simulink model "AEBsystem"  (R2024a)
settings: Solver=VariableStepAuto  StartTime=0.0  StopTime=15  RelTol=1e-3
InitFcn:
  | INITAEB
values from neighbouring files (symbols this model uses):
  conducteurActive_var = Simulink.Parameter    [INITAEB.m]
  decelConducteur = 1.5    [INITAEB.m]
  FFORT_decel = 5.0    (= 5)    [INITAEB.m]
  headwayOffset = 1.0    (= 1)    [INITAEB.m]
  PB1_decel = 1.8    [INITAEB.m]
  PB2_decel = 3.2    [INITAEB.m]
  timeMargin = 0.3    [INITAEB.m]
libraries: simulink x4, sim3dautolib x2, sim3dlib x1
(part 2 of 2)

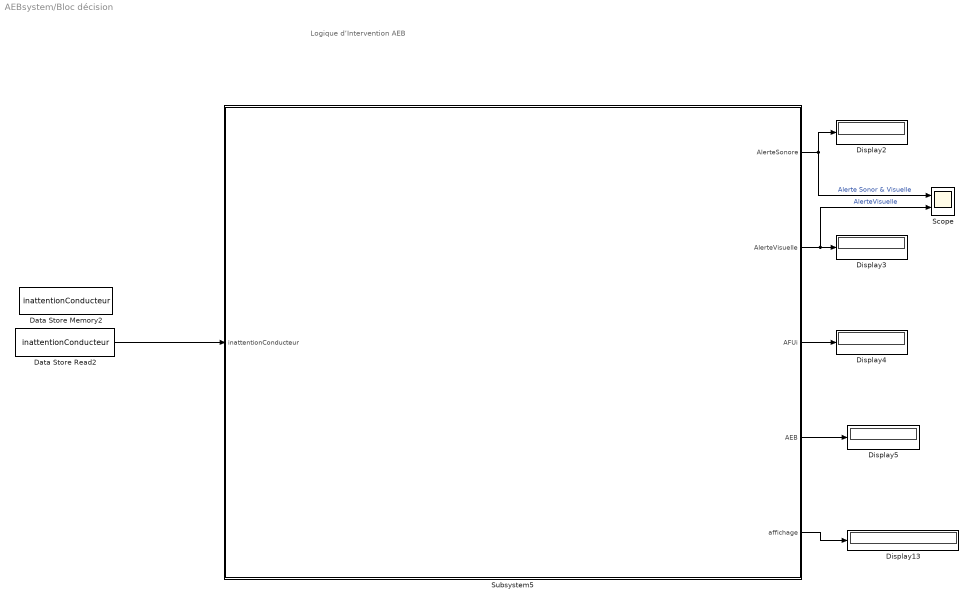
== system AEBsystem/Bloc décision  ==
  note: Logique d’Intervention AEB
  Data Store Memory2 : DataStoreMemory  DataStoreName=inattentionConducteur  WriteAfterWriteMsg=warning  ShowAdditionalParam=off
  Data Store Read2 : DataStoreRead  DataStoreName=inattentionConducteur  IndexOptions=Index vector (dialog)  Indices=1  OutputSizes=1
  Display{2..5,13} (5 alike) : Display
  Scope : Scope  NumInputPorts=2
  Subsystem5 : Subsystem
  wires:
  Subsystem5/1(AlerteSonore) -> Display2/1, Scope/1  "Alerte Sonor & Visuelle"
  Subsystem5/3(AFUi) -> Display4/1
  Subsystem5/2(AlerteVisuelle) -> Scope/2, Display3/1  "AlerteVisuelle"
  Data Store Read2/1 -> Subsystem5/1(inattentionConducteur)
  Subsystem5/4(AEB) -> Display5/1
  Subsystem5/5(affichage) -> Display13/1

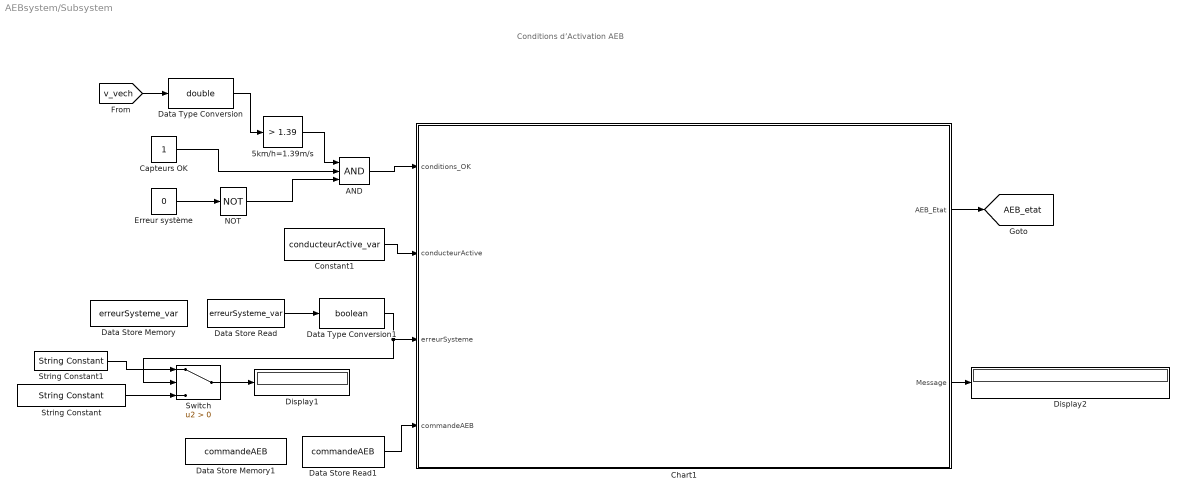
== system AEBsystem/Subsystem ==
  note: Conditions d’Activation AEB
  5km/h=1.39m/s : simulink/Logic and Bit Operations/Compare To Constant  relop=>  const=1.39  OutDataTypeStr=uint8
  AND : Logic  Inputs=3  IconShape=distinctive  AllPortsSameDT=off  OutDataTypeStr=boolean
  Capteurs OK : Constant
  Chart1 : Stateflow chart  TreatAsAtomicUnit=on
  Constant1 : Constant  Value=conducteurActive_var
  Data Store Memory : DataStoreMemory  DataStoreName=erreurSysteme_var  WriteAfterWriteMsg=warning  ShowAdditionalParam=off
  Data Store Memory1 : DataStoreMemory  DataStoreName=commandeAEB  WriteAfterWriteMsg=warning  InitialValue=1  ShowAdditionalParam=off
  Data Store Read : DataStoreRead  DataStoreName=erreurSysteme_var  IndexOptions=Index vector (dialog)  Indices=1  OutputSizes=1
  Data Store Read1 : DataStoreRead  DataStoreName=commandeAEB  IndexOptions=Index vector (dialog)  Indices=1  OutputSizes=1
  Data Type Conversion : DataTypeConversion  OutDataTypeStr=double  SaturateOnIntegerOverflow=off  RndMeth=Floor
  Data Type Conversion1 : DataTypeConversion  OutDataTypeStr=boolean  SaturateOnIntegerOverflow=off  RndMeth=Floor
  Display1 : Display
  Display2 : Display
  Erreur système : Constant  Value=0
  NOT : Logic  Operator=NOT  IconShape=distinctive  AllPortsSameDT=off  OutDataTypeStr=boolean
  String Constant : StringConstant  String=Pas_en_panne
  String Constant1 : StringConstant  String=en_panne
  Switch : Switch  Criteria=u2 > Threshold  SaturateOnIntegerOverflow=off  InputSameDT=off
  tag scope: AEB_etat=global
  wires:
  Data Store Read/1 -> Data Type Conversion1/1
  Data Type Conversion/1 -> 5km/h=1.39m/s/1
  NOT/1 -> AND/3
  AND/1 -> Chart1/1(conditions_OK)
  String Constant/1 -> Switch/3
  5km/h=1.39m/s/1 -> AND/1
  Capteurs OK/1 -> AND/2
  String Constant1/1 -> Switch/1
  Constant1/1 -> Chart1/2(conducteurActive)
  Data Type Conversion1/1 -> Switch/2, Chart1/3(erreurSysteme)
  Switch/1 -> Display1/1
  Data Store Read1/1 -> Chart1/4(commandeAEB)
  Chart1/2(Message) -> Display2/1
  Erreur système/1 -> NOT/1
  Chart1/1(AEB_Etat) -> [AEB_etat]
  [v_vech] -> Data Type Conversion/1

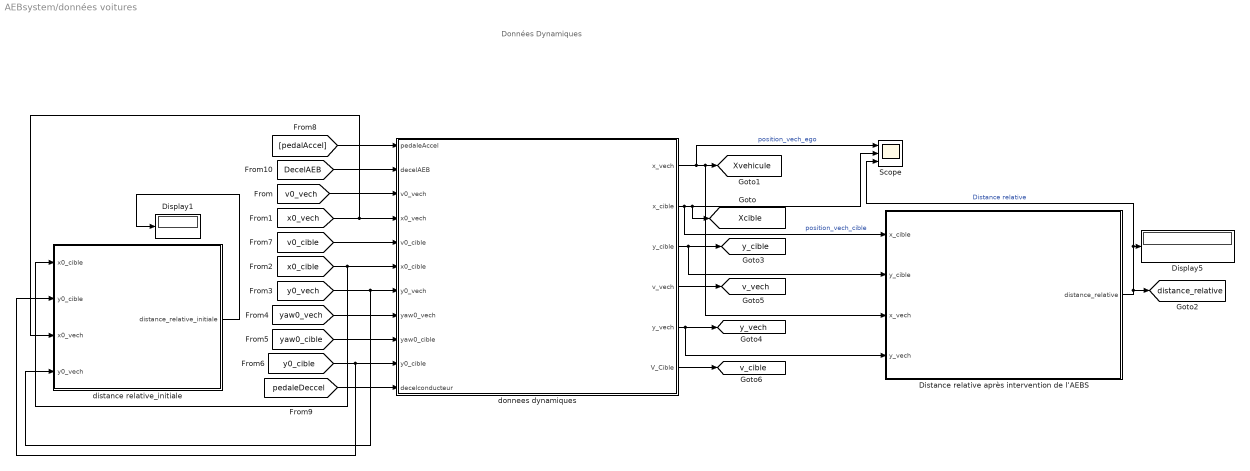
== system AEBsystem/données voitures ==
  note: Données Dynamiques
  Display1 : Display
  Display5 : Display
  Distance relative après intervention de l’AEBS : Subsystem
  Scope : Scope  NumInputPorts=3
  distance relative_initiale : Subsystem
  "donnees dynamiques " : Subsystem
  tag scope: Xcible=global, Xvehicule=global, distance_relative=global, v_cible=global, v_vech=global, y_cible=global, y_vech=global
  wires:
  "donnees dynamiques "/2(x_cible) -> Distance relative après intervention de l’AEBS/1(x_cible), Scope/2, [Xcible]  "position_vech_cible"
  Distance relative après intervention de l’AEBS/1(distance_relative) -> [distance_relative], Scope/3, Display5/1  "Distance relative"
  [v0_vech] -> "donnees dynamiques "/3(v0_vech)
  [x0_cible] -> "donnees dynamiques "/6("x0_cible "), distance relative_initiale/1(x0_cible)
  [y0_vech] -> distance relative_initiale/4(y0_vech), "donnees dynamiques "/7(y0_vech)
  [yaw0_vech] -> "donnees dynamiques "/8(yaw0_vech)
  [yaw0_cible] -> "donnees dynamiques "/9(yaw0_cible)
  "donnees dynamiques "/4(v_vech) -> [v_vech]
  [x0_vech] -> "donnees dynamiques "/4(x0_vech), distance relative_initiale/3(x0_vech)
  [y0_cible] -> "donnees dynamiques "/10("y0_cible "), distance relative_initiale/2(y0_cible)
  distance relative_initiale/1(distance_relative_initiale) -> Display1/1
  [pedalAccel] -> "donnees dynamiques "/1(pedaleAccel)
  [pedaleDeccel] -> "donnees dynamiques "/11(decelconducteur)
  [DecelAEB] -> "donnees dynamiques "/2(decelAEB)
  "donnees dynamiques "/6(V_Cible) -> [v_cible]
  [v0_cible] -> "donnees dynamiques "/5(v0_cible)
  "donnees dynamiques "/5(y_vech) -> Distance relative après intervention de l’AEBS/4(y_vech), [y_vech]
  "donnees dynamiques "/3(y_cible) -> Distance relative après intervention de l’AEBS/2(y_cible), [y_cible]
  "donnees dynamiques "/1(x_vech) -> Scope/1, Distance relative après intervention de l’AEBS/3(x_vech), [Xvehicule]  "position_vech_ego"

== system AEBsystem/voiture_cible ==
  Constant1 : Constant  Value=y0_cible
  Constant2 : Constant  Value=v0_cible
  Constant3 : Constant  Value=yaw0_cible
  Constant6 : Constant  Value=x0_cible
  Out1 : Outport
  Out2 : Outport  Port=2
  Out3 : Outport  Port=3
  Out4 : Outport  Port=4
  wires:
  Constant3/1 -> Out4/1
  Constant1/1 -> Out2/1
  Constant2/1 -> Out3/1
  Constant6/1 -> Out1/1

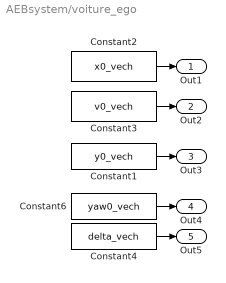
== system AEBsystem/voiture_ego ==
  Constant1 : Constant  Value=y0_vech  OutDataTypeStr=double
  Constant2 : Constant  Value=x0_vech  OutDataTypeStr=double
  Constant3 : Constant  Value=v0_vech  OutDataTypeStr=double
  Constant4 : Constant  Value=delta_vech
  Constant6 : Constant  Value=yaw0_vech
  Out1 : Outport
  Out2 : Outport  Port=2
  Out3 : Outport  Port=3
  Out4 : Outport  Port=4
  Out5 : Outport  Port=5
  wires:
  Constant1/1 -> Out3/1
  Constant6/1 -> Out4/1
  Constant3/1 -> Out2/1
  Constant2/1 -> Out1/1
  Constant4/1 -> Out5/1

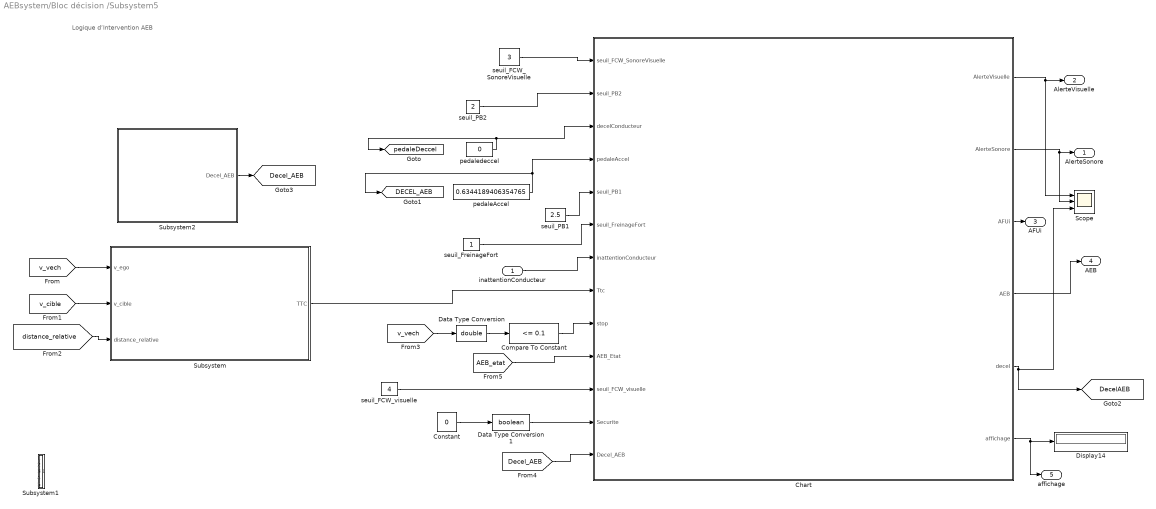
== system AEBsystem/Bloc décision /Subsystem5 ==
  note: Logique d’Intervention AEB
  inattentionConducteur : Inport
  Chart : Stateflow chart  TreatAsAtomicUnit=on
      settings: PortSchema="{\"entries\":[{\"content\":{\"sides\":[{\"content\":{\"connectorIds\":[\"In1\",\"In2\",\"In3\",\"In6\",\"In4\",\"In5\",\"In7\",\"In8\",\"In9\",\"In10\",\"In11\",\"In12\",\"In13\"]},\"type\":\"ConnectorPlacement.EquallySpacedRectSide\",\"uuid\":\"ac4113fa-98ee-4c5c-b1a8-e2b3c82a8f48\"},{\"content\":{\"connectorIds\":[\"Out1\",\"Out2\",\"Out3\",\"Out4\",\"Out5\",\"Out6\"],\"side\":\"RIGHT\"},\"type\":\"ConnectorPlacement.EquallySpacedRectSide\",\"uuid\":\"41eea1f7-be6c-483d-8938-9d006cfb1316\"},{\"content\":{\"side\":\"TOP\"},\"type\":\"ConnectorPlacement.EquallySpacedRectSide\",\"uuid\":\"fe521d2a-0fb3-48e4-9d91-7764065f447c\"}]},\"type\":\"ConnectorPlacement.EquallySpacedConnector\",\"uuid\":\"e83fd15b-6ef2-462f-822e-3091780eb47e\"}],\"packageUris\":[\"http://schema.mathworks.com/mf0/Connector/R2020b\"],\"version\":\"1.0\"}"
  Compare To Constant : simulink/Logic and Bit Operations/Compare To Constant  relop=<=  const=0.1  OutDataTypeStr=boolean
  Constant : Constant  Value=0
  Data Type Conversion : DataTypeConversion  OutDataTypeStr=double  SaturateOnIntegerOverflow=off  RndMeth=Floor
  Data Type Conversion1 : DataTypeConversion  OutDataTypeStr=boolean  SaturateOnIntegerOverflow=off  RndMeth=Floor
  Display14 : Display
  Scope : Scope  NumInputPorts=3
  Subsystem : Subsystem
  Subsystem1 : Subsystem
  Subsystem2 : Subsystem
  pedaleAccel : Constant  Value=0.6344189406354765
  pedaledeccel : Constant  Value=0
  seuil_FCW_SonoreVisuelle : Constant  Value=3
  seuil_FCW_visuelle : Constant  Value=4
  seuil_FreinageFort : Constant
  seuil_PB1 : Constant  Value=2.5
  seuil_PB2 : Constant  Value=2
  AlerteSonore : Outport
  AlerteVisuelle : Outport  Port=2
  AFUi : Outport  Port=3
  AEB : Outport  Port=4
  affichage : Outport  Port=5
  tag scope: DECEL_AEB=global, DecelAEB=global, Decel_AEB=global, pedaleDeccel=global
  wires:
  Compare To Constant/1 -> Chart/9(stop)
  Data Type Conversion/1 -> Compare To Constant/1
  Chart/1(AlerteVisuelle) -> AlerteVisuelle/1, Scope/1
  Chart/2(AlerteSonore) -> Scope/2, AlerteSonore/1
  Chart/3(AFUi) -> AFUi/1
  pedaledeccel/1 -> Chart/3(decelConducteur), [pedaleDeccel]
  inattentionConducteur/1 -> Chart/7(inattentionConducteur)
  Chart/4(AEB) -> AEB/1
  Chart/6(affichage) -> affichage/1, Display14/1
  Constant/1 -> Data Type Conversion1/1
  Data Type Conversion1/1 -> Chart/12(Securite)
  pedaleAccel/1 -> [DECEL_AEB], Chart/6(pedaleAccel)
  [v_vech] -> Subsystem/1(v_ego)
  [v_cible] -> Subsystem/2(v_cible)
  [distance_relative] -> Subsystem/3(distance_relative)
  [v_vech] -> Data Type Conversion/1
  Subsystem/1(TTC) -> Chart/8(Ttc)
  [AEB_etat] -> Chart/10(AEB_Etat)
  seuil_FreinageFort/1 -> Chart/5(seuil_FreinageFort)
  seuil_FCW_visuelle/1 -> Chart/11(seuil_FCW_visuelle)
  seuil_FCW_SonoreVisuelle/1 -> Chart/1(seuil_FCW_SonoreVisuelle)
  seuil_PB1/1 -> Chart/4(seuil_PB1)
  seuil_PB2/1 -> Chart/2(seuil_PB2)
  Subsystem2/1(Decel_AEB) -> [Decel_AEB]
  [Decel_AEB] -> Chart/13(Decel_AEB)
  Chart/5(decel) -> [DecelAEB], Scope/3

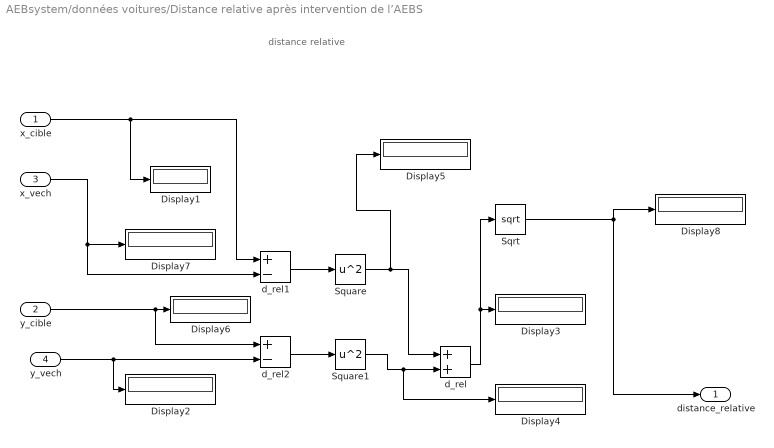
== system AEBsystem/données voitures/Distance relative après intervention de l’AEBS ==
  note: distance relative
  x_cible : Inport
  y_cible : Inport  Port=2
  x_vech : Inport  Port=3
  y_vech : Inport  Port=4
  Display{1..8} (8 alike) : Display
  Sqrt : Sqrt
  Square : Math  Operator=square
  Square1 : Math  Operator=square
  d_rel : Sum  OutDataTypeStr=double
  d_rel1 : Sum  Inputs=+-  OutDataTypeStr=double
  d_rel2 : Sum  Inputs=+-  OutDataTypeStr=double
  distance_relative : Outport
  wires:
  d_rel2/1 -> Square1/1
  Square1/1 -> Display4/1, d_rel/2
  x_vech/1 -> d_rel1/2, Display7/1
  d_rel/1 -> Sqrt/1, Display3/1
  y_vech/1 -> Display2/1, d_rel2/2
  Square/1 -> Display5/1, d_rel/1
  d_rel1/1 -> Square/1
  Sqrt/1 -> distance_relative/1, Display8/1
  y_cible/1 -> d_rel2/1, Display6/1
  x_cible/1 -> Display1/1, d_rel1/1

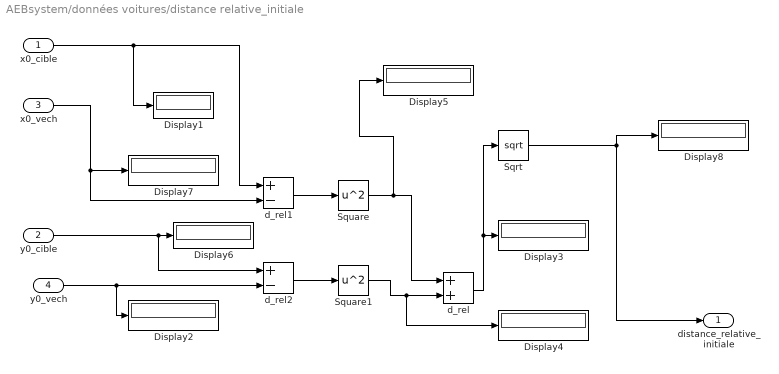
== system AEBsystem/données voitures/distance relative_initiale ==
  x0_cible : Inport
  y0_cible : Inport  Port=2
  x0_vech : Inport  Port=3
  y0_vech : Inport  Port=4
  Display{1..8} (8 alike) : Display
  Sqrt : Sqrt
  Square : Math  Operator=square
  Square1 : Math  Operator=square
  d_rel : Sum  OutDataTypeStr=double
  d_rel1 : Sum  Inputs=+-  OutDataTypeStr=double
  d_rel2 : Sum  Inputs=+-  OutDataTypeStr=double
  distance_relative_initiale : Outport
  wires:
  d_rel2/1 -> Square1/1
  Square1/1 -> Display4/1, d_rel/2
  x0_vech/1 -> d_rel1/2, Display7/1
  d_rel/1 -> Sqrt/1, Display3/1
  y0_vech/1 -> Display2/1, d_rel2/2
  Square/1 -> Display5/1, d_rel/1
  d_rel1/1 -> Square/1
  Sqrt/1 -> distance_relative_initiale/1, Display8/1
  y0_cible/1 -> d_rel2/1, Display6/1
  x0_cible/1 -> Display1/1, d_rel1/1

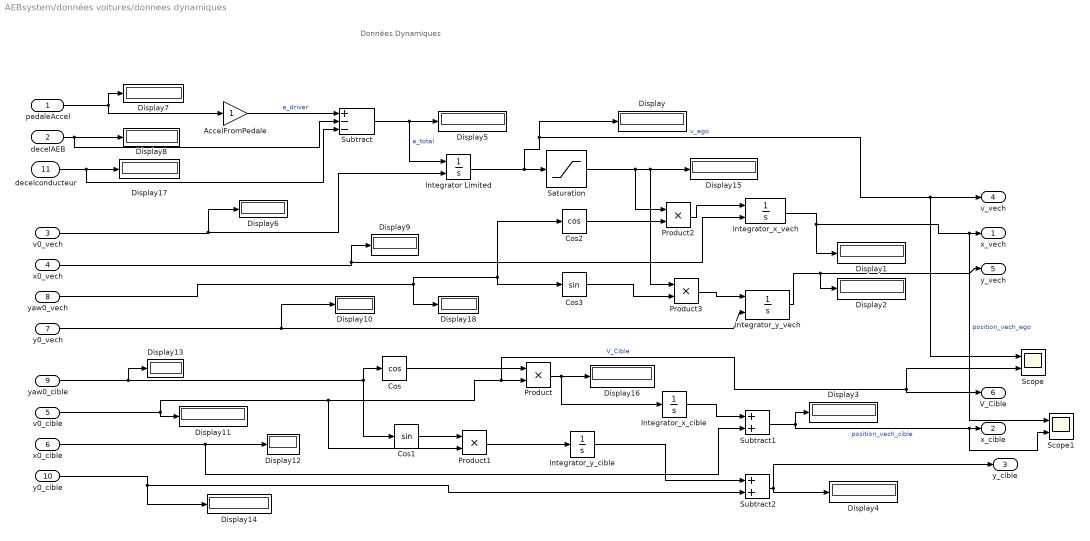
== system AEBsystem/données voitures/donnees dynamiques  ==
  note: Données Dynamiques
  pedaleAccel : Inport
  decelAEB : Inport  Port=2
  v0_vech : Inport  Port=3
  x0_vech : Inport  Port=4
  v0_cible : Inport  Port=5
  "x0_cible " : Inport  Port=6
  y0_vech : Inport  Port=7
  yaw0_vech : Inport  Port=8
  yaw0_cible : Inport  Port=9
  "y0_cible " : Inport  Port=10
  decelconducteur : Inport  Port=11
  AccelFromPedale : Gain
  Cos : Trigonometry  Operator=cos
  Cos1 : Trigonometry
  Cos2 : Trigonometry  Operator=cos
  Cos3 : Trigonometry
  Display{,1..18} (19 alike) : Display
  Integrator Limited : Integrator  InitialConditionSource=external  LimitOutput=on  UpperSaturationLimit=80  LowerSaturationLimit=0
  Integrator_x_cible : Integrator  LimitOutput=on  UpperSaturationLimit=500  LowerSaturationLimit=-50
  Integrator_x_vech : Integrator  InitialConditionSource=external  LimitOutput=on  UpperSaturationLimit=500  LowerSaturationLimit=-50
  Integrator_y_cible : Integrator  LimitOutput=on  UpperSaturationLimit=500  LowerSaturationLimit=-50
  Integrator_y_vech : Integrator  InitialConditionSource=external  LimitOutput=on  UpperSaturationLimit=500  LowerSaturationLimit=-50
  Product{,1..3} (4 alike) : Product
  Saturation : Saturate  UpperLimit=200  LowerLimit=0
  Scope : Scope  NumInputPorts=2
  Scope1 : Scope  NumInputPorts=2
  Subtract : Sum  Inputs=+--
  Subtract1 : Sum
  Subtract2 : Sum
  x_vech : Outport
  x_cible : Outport  Port=2
  y_cible : Outport  Port=3
  v_vech : Outport  Port=4
  y_vech : Outport  Port=5
  V_Cible : Outport  Port=6
  wires:
  Subtract/1 -> Integrator Limited/1, Display5/1  "a_total"
  decelAEB/1 -> Subtract/2, Display8/1
  pedaleAccel/1 -> AccelFromPedale/1, Display7/1
  AccelFromPedale/1 -> Subtract/1  "a_driver"
  v0_vech/1 -> Display6/1, Integrator Limited/2
  x0_vech/1 -> Integrator_x_vech/2, Display9/1
  v0_cible/1 -> Display11/1, V_Cible/1, Scope/2, Product/2, Product1/2  "V_Cible"
  "x0_cible "/1 -> Subtract1/2, Display12/1
  Cos/1 -> Product/1
  Product/1 -> Integrator_x_cible/1, Display16/1
  Integrator_x_cible/1 -> Subtract1/1
  yaw0_cible/1 -> Display13/1, Cos/1, Cos1/1
  Cos1/1 -> Product1/1
  Product1/1 -> Integrator_y_cible/1
  yaw0_vech/1 -> Cos2/1, Cos3/1, Display18/1
  Cos2/1 -> Product2/2
  Product2/1 -> Integrator_x_vech/1
  Cos3/1 -> Product3/2
  Product3/1 -> Integrator_y_vech/1
  Integrator Limited/1 -> Saturation/1, Display/1, Scope/1, v_vech/1  "v_ego"
  Integrator_y_vech/1 -> y_vech/1, Display2/1
  y0_vech/1 -> Display10/1, Integrator_y_vech/2
  Saturation/1 -> Product2/1, Product3/1, Display15/1
  Subtract2/1 -> y_cible/1, Display4/1
  Integrator_y_cible/1 -> Subtract2/1
  decelconducteur/1 -> Subtract/3, Display17/1
  "y0_cible "/1 -> Display14/1, Subtract2/2
  Subtract1/1 -> Scope1/2, x_cible/1, Display3/1  "position_vech_cible"
  Integrator_x_vech/1 -> Display1/1, Scope1/1, x_vech/1  "position_vech_ego"

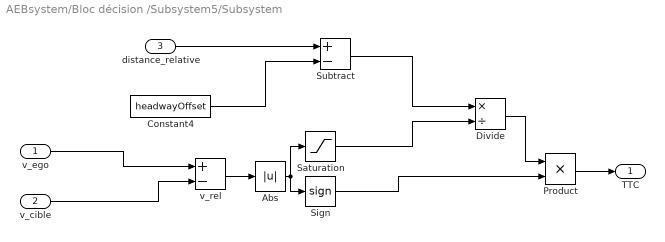
== system AEBsystem/Bloc décision /Subsystem5/Subsystem ==
  v_ego : Inport
  v_cible : Inport  Port=2
  distance_relative : Inport  Port=3
  Abs : Abs  OutDataTypeStr=double  SaturateOnIntegerOverflow=off
  Constant4 : Constant  Value=headwayOffset
  Divide : Product  Inputs=*/
  Product : Product
  Saturation : Saturate  UpperLimit=100
  Sign : Signum
  Subtract : Sum  Inputs=+-  OutDataTypeStr=double
  v_rel : Sum  Inputs=+-  OutDataTypeStr=double
  TTC : Outport  OutDataTypeStr=double
  wires:
  Saturation/1 -> Divide/2
  Sign/1 -> Product/2
  v_ego/1 -> v_rel/1
  Divide/1 -> Product/1
  distance_relative/1 -> Subtract/1
  v_cible/1 -> v_rel/2
  v_rel/1 -> Abs/1
  Abs/1 -> Sign/1, Saturation/1
  Product/1 -> TTC/1
  Subtract/1 -> Divide/1
  Constant4/1 -> Subtract/2

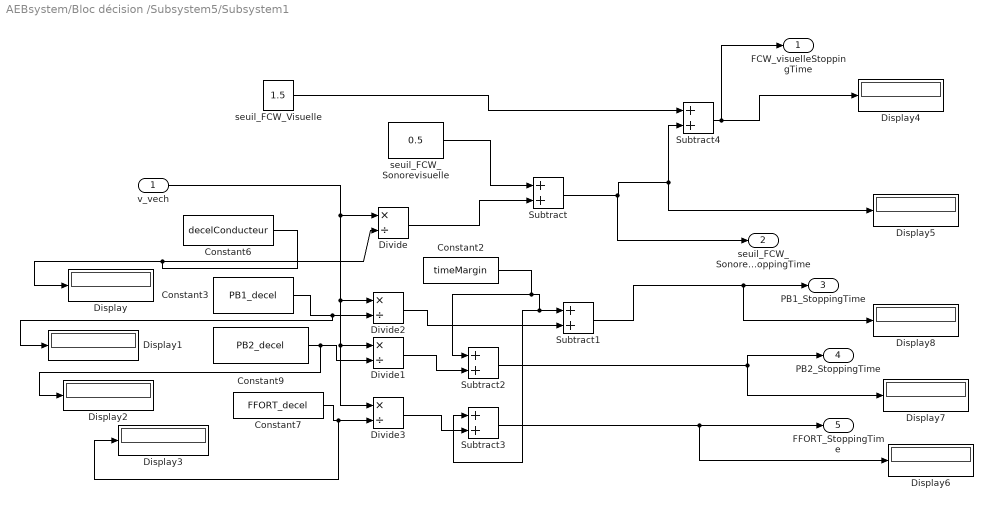
== system AEBsystem/Bloc décision /Subsystem5/Subsystem1 ==
  v_vech : Inport
  Constant2 : Constant  Value=timeMargin
  Constant3 : Constant  Value=PB1_decel
  Constant6 : Constant  Value=decelConducteur
  Constant7 : Constant  Value=FFORT_decel  OutDataTypeStr=double
  Constant9 : Constant  Value=PB2_decel  OutDataTypeStr=double
  Display{,1..8} (9 alike) : Display
  Divide{,1..3} (4 alike) : Product  Inputs=*/
  Subtract{,1..4} (5 alike) : Sum
  seuil_FCW_Sonorevisuelle : Constant  Value=0.5  OutDataTypeStr=double
  seuil_FCW_Visuelle : Constant  Value=1.5  OutDataTypeStr=double
  FCW_visuelleStoppingTime : Outport  OutDataTypeStr=double
  seuil_FCW_SonoreVisuelleStoppingTime : Outport  Port=2  OutDataTypeStr=double
  PB1_StoppingTime : Outport  Port=3  OutDataTypeStr=double
  PB2_StoppingTime : Outport  Port=4  OutDataTypeStr=double
  FFORT_StoppingTime : Outport  Port=5  OutDataTypeStr=double
  wires:
  Subtract2/1 -> Display7/1, PB2_StoppingTime/1
  seuil_FCW_Sonorevisuelle/1 -> Subtract/1
  Divide/1 -> Subtract/2
  Divide1/1 -> Subtract2/2
  Divide2/1 -> Subtract1/2
  Constant7/1 -> Display3/1, Divide3/2
  Subtract4/1 -> Display4/1, FCW_visuelleStoppingTime/1
  v_vech/1 -> Divide1/1, Divide3/1, Divide2/1, Divide/1
  Divide3/1 -> Subtract3/2
  Constant3/1 -> Display1/1, Divide2/2
  Subtract1/1 -> Display8/1, PB1_StoppingTime/1
  Subtract/1 -> seuil_FCW_SonoreVisuelleStoppingTime/1, Display5/1, Subtract4/2
  Constant9/1 -> Display2/1, Divide1/2
  Subtract3/1 -> Display6/1, FFORT_StoppingTime/1
  Constant2/1 -> Subtract1/1, Subtract3/1, Subtract2/1
  Constant6/1 -> Divide/2, Display/1
  seuil_FCW_Visuelle/1 -> Subtract4/1

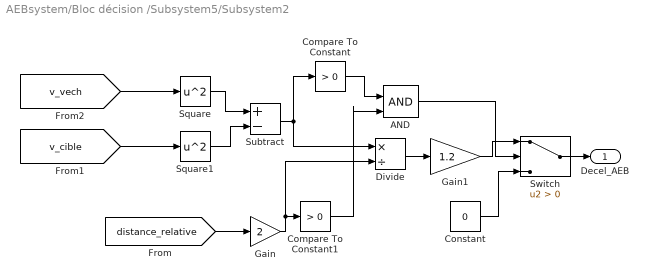
== system AEBsystem/Bloc décision /Subsystem5/Subsystem2 ==
  AND : Logic  IconShape=distinctive  AllPortsSameDT=off  OutDataTypeStr=boolean
  Compare To Constant : simulink/Logic and Bit Operations/Compare To Constant  relop=>  const=0  OutDataTypeStr=boolean
  Compare To Constant1 : simulink/Logic and Bit Operations/Compare To Constant  relop=>  const=0  OutDataTypeStr=boolean
  Constant : Constant  Value=0
  Divide : Product  Inputs=*/
  Gain : Gain  Gain=2
  Gain1 : Gain  Gain=1.2
  Square : Math  Operator=square
  Square1 : Math  Operator=square
  Subtract : Sum  Inputs=+-
  Switch : Switch  Criteria=u2 > Threshold  SaturateOnIntegerOverflow=off  InputSameDT=off
  Decel_AEB : Outport
  wires:
  [v_vech] -> Square/1
  [v_cible] -> Square1/1
  Square/1 -> Subtract/1
  Square1/1 -> Subtract/2
  [distance_relative] -> Gain/1
  Divide/1 -> Gain1/1
  Subtract/1 -> Compare To Constant/1, Divide/1
  Compare To Constant/1 -> AND/1
  Gain/1 -> Divide/2, Compare To Constant1/1
  Switch/1 -> Decel_AEB/1
  Constant/1 -> Switch/3
  Compare To Constant1/1 -> AND/2
  AND/1 -> Switch/2
  Gain1/1 -> Switch/1

== stateflow chart AEBsystem/Subsystem/Chart1 ==
  state stateInhibe
    entry:
    AEB_Etat = 0;
    Message = "Fonction inhibee";
  state stateDeselectionne
    entry:
    AEB_Etat = 0;
    Message = "Deselectionne par le conducteur";
  state stateSelectionne
    entry:
    AEB_Etat = 0;
    Message = "Selectionne - attente activation";
  state stateDesactive
    entry:
    AEB_Etat = 1;
    Message = "AEB desactive - conditions non remplies";
  state stateActive
    entry:
    AEB_Etat = 2;
    Message = "AEB active - freinage automatique possible";
  state stateEn_Panne
    entry:
    AEB_Etat = 0;
    Message = "Erreur systeme - Fonction en panne";
  (default) -> stateInhibe
  stateDesactive -> stateInhibe [order 3] : [commandeAEB == false]
  stateSelectionne -> stateInhibe [order 4] : [commandeAEB == false]
  stateActive -> stateInhibe [order 3] : [commandeAEB == false]
  stateInhibe -> stateDeselectionne
  stateDeselectionne -> stateEn_Panne [order 2] : [erreurSysteme == true]
  stateDeselectionne -> stateSelectionne [order 1] : [commandeAEB == true && conducteurActive == true]
  stateSelectionne -> stateDeselectionne [order 1] : [conducteurActive == false]
  stateSelectionne -> stateEn_Panne [order 3] : [erreurSysteme == true]
  stateSelectionne -> stateDesactive [order 2] : [conditions_OK == false]
  stateSelectionne -> stateActive [order 5]
  stateDesactive -> stateEn_Panne [order 2] : [erreurSysteme == true]
  stateActive -> stateDesactive [order 1] : [conditions_OK == false ]
  stateDesactive -> stateActive [order 1] : [conditions_OK == true]
  stateActive -> stateEn_Panne [order 2] : [erreurSysteme == true]
  data: conditions_OK input boolean; conducteurActive input boolean; erreurSysteme input boolean; AEB_Etat output int8; Message output string; commandeAEB input boolean

== stateflow chart AEBsystem/Bloc décision /Subsystem5/Chart ==
  state Stop_fix
    entry:
    AEB = 0;
    AFUi = false;
    AlerteSonore = false;
    AlerteVisuelle = false;
    decel = 0;
    affichage = "Stop !";
  state Default_
    entry:
    AEB = 0;
    AFUi = false;
    AlerteSonore = false;
    AlerteVisuelle = false;
    decel = 0;
    affichage = "Systeme inactif";
  state FCW_SonoreVisuelle
    entry:
    AEB = 0;
    AlerteSonore = true;
    AlerteVisuelle = true;
    AFUi = false;
    decel = 0;
    affichage = "freinez !";
  state FCW_Visuelle
    entry:
    AEB = 0;
    AFUi = false;
    AlerteSonore = false;
    AlerteVisuelle = true;
    decel = 0;
    affichage = "Vehicule proche ! ";
  state Assistance
    entry:
    AEB = 1;
    AFUi = true;
    AlerteSonore = false;
    AlerteVisuelle = false
    decel = 3.0;
    affichage = "AFUi active/decel = 3";
  state PB1
    entry:
    AEB = 2;
    AlerteSonore = false;
    AlerteVisuelle = false;
    AFUi = false;
    decel = 3.8;
    affichage = "PB1 active/decel = 3.8";
  state Freinage
    entry:
    AEB = 4;
    AlerteSonore = false;
    AlerteVisuelle = false;
    AFUi = false;
    decel = Decel_AEB;
    affichage = "FreinageFort ";
  state PB2
    entry:
    AEB = 3;
    AlerteSonore = false
    AlerteVisuelle = false
    AFUi = false;
    decel = 5.8;
    affichage = "PB2 active/decel = 5.8";
  (default) -> Default_
  Stop_fix -> Default_ : [Securite ==1 ]
  FCW_SonoreVisuelle -> Stop_fix [order 1] : [stop == true]
  Assistance -> Stop_fix [order 1] : [decelConducteur >= 4.0  ]
  Freinage -> Stop_fix : [stop == true]
  FCW_Visuelle -> Stop_fix [order 1] : [stop == true]
  PB2 -> Stop_fix [order 2] : [stop == true]
  Default_ -> FCW_Visuelle : [  AEB_Etat == 2 && ( all(seuil_FCW_visuelle > abs(Ttc)) && all(inattentionConducteur == false) && all(pedaleAccel < 0.8) || all(inattentionConducteur == true) && all(pedaleAccel > 0.8) && all(seuil_FCW_visuelle > abs(Ttc)))]
  PB1 -> Stop_fix [order 2] : [stop == true]
  FCW_Visuelle -> FCW_SonoreVisuelle [order 2] : [  all(seuil_FCW_SonoreVisuelle > abs(Ttc)) ]
  FCW_SonoreVisuelle -> Assistance [order 3] : [decelConducteur >= 3.5 && (all(abs(Ttc) > seuil_PB1)) ]
  FCW_SonoreVisuelle -> PB1 [order 2] : [ (all(abs(Ttc) < seuil_PB1))  ]
  Assistance -> PB1 [order 2] : [ decelConducteur < 3.5 || all(abs(Ttc) < seuil_PB1) ]
  PB1 -> PB2 [order 1] : [( all(seuil_PB2 > abs(Ttc)))]
  PB2 -> Freinage [order 1] : [(all(abs(Ttc) < seuil_FreinageFort)) ]
  data: seuil_FCW_SonoreVisuelle input double size=1; seuil_PB2 input double size=1; decelConducteur input double size=1; seuil_PB1 input double size=1; seuil_FreinageFort input double size=1; pedaleAccel input double size=1; inattentionConducteur input boolean size=1; Ttc input double size=1; stop input boolean size=1; AlerteVisuelle output boolean size=1; AlerteSonore output boolean size=1; AFUi output boolean size=1; AEB output double size=1; decel output double size=1; AEB_Etat input int8; seuil_FCW_visuelle input; affichage output string; Securite input boolean; Decel_AEB input
